simulink library "MFMdl7"  (Simulink 8.8)
settings: Solver=VariableStepAuto  StartTime=0.0  StopTime=10.0  RelTol=1e-3
libraries: simulink x3
settings Model: Creator=viett  LastModifiedBy=viett

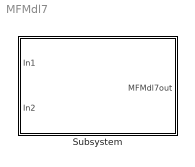
== system MFMdl7 ==
  Subsystem : Subsystem

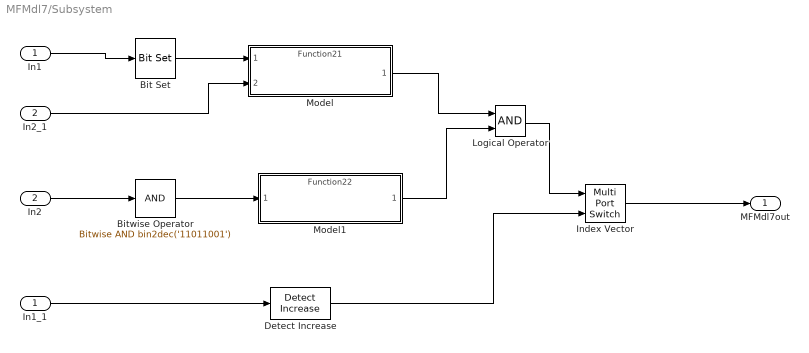
== system MFMdl7/Subsystem ==
  In1 : Inport
  In2 : Inport  Port=2
  Bit Set : simulink/Logic and Bit Operations/Bit Set  iBit=0
  Bitwise Operator : simulink/Logic and Bit Operations/Bitwise Operator  logicop=AND  UseBitMask=on  BitMask=bin2dec('11011001')  BitMaskRealWorld=Stored Integer
  Detect Increase : simulink/Logic and Bit Operations/Detect Increase  vinit=0.0  OutDataTypeStr=boolean
  In1_1 : InportShadow
  In2_1 : InportShadow  Port=2
  Index Vector : MultiPortSwitch  DataPortOrder=Zero-based contiguous  Inputs=1  zeroidx=on
  Logical Operator : Logic  AllPortsSameDT=off  OutDataTypeStr=boolean
  Model : ModelReference  ModelNameDialog=Function21.slx  SimulationMode=Normal  ModelReferenceVersion=1.3
  Model1 : ModelReference  ModelNameDialog=Function22.slx  SimulationMode=Normal  ModelReferenceVersion=1.3
  MFMdl7out : Outport
  wires:
  Logical Operator/1 -> Index Vector/1
  Model1/1 -> Logical Operator/2
  Bit Set/1 -> Model/1
  In1_1/1 -> Detect Increase/1
  In2/1 -> Bitwise Operator/1
  In2_1/1 -> Model/2
  Index Vector/1 -> MFMdl7out/1
  Model/1 -> Logical Operator/1
  Detect Increase/1 -> Index Vector/2
  Bitwise Operator/1 -> Model1/1
  In1/1 -> Bit Set/1
